simulink model "SixDOFFINAL"  (R2025a)
settings: Solver=FixedStepAuto  StartTime=0.0  StopTime=10  FixedStep=0.001  RelTol=1e-8
PreLoadFcn:
  | P = rocketConfigEuler();
  | assignin('base','P',P);
settings Model: Creator=olive  LastModifiedBy=olivermcnaughton
settings DebuggingCC: UnderSpecifiedDimensionMsg=warning

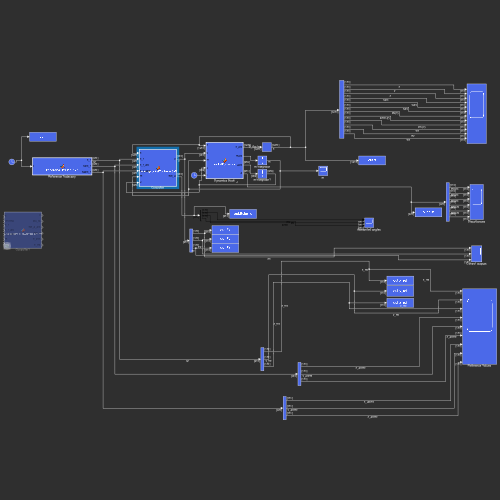
[thumbnail: Simulink's stored preview of the top-level diagram]
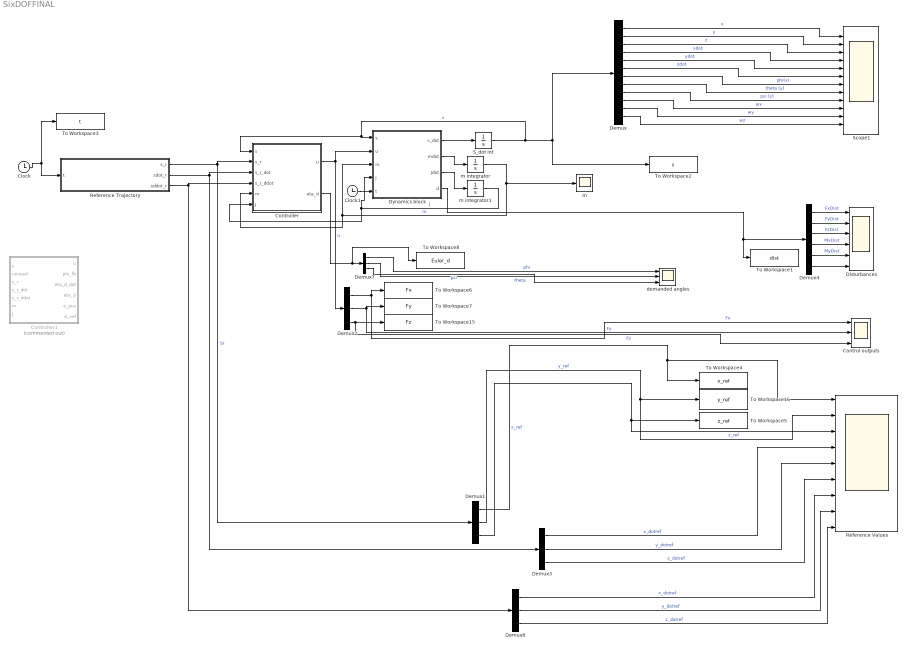
== system SixDOFFINAL ==
  Clock : Clock
  Clock1 : Clock
  Control outputs : Scope  NumInputPorts=3
      settings: ActiveDisplayYMinimum=-27.646396569156394  ActiveDisplayYMaximum=103.07182184101738  DataLoggingVariableName=ScopeData3
  Controller : MATLAB Function  TreatAsAtomicUnit=on
  Controller1 : MATLAB Function  Commented=on  TreatAsAtomicUnit=on
  Demux : Demux  Outputs=12
  Demux{1..3,7..8} (5 alike) : Demux  Outputs=3
  Demux4 : Demux  Outputs=6
  Disturbances : Scope  NumInputPorts=6
      settings: ActiveDisplayYMinimum=-1  ActiveDisplayYMaximum=1
  Dynamics block : MATLAB Function  TreatAsAtomicUnit=on
  Reference Trajectory : MATLAB Function  TreatAsAtomicUnit=on
  Reference Values : Scope  NumInputPorts=9
      settings: ActiveDisplayYMinimum=-0.49999999999999989  ActiveDisplayYMaximum=4.5  DataLoggingVariableName=ScopeData4
  S_dot int : Integrator  InitialCondition=P.init.stateDot
  Scope1 : Scope  NumInputPorts=12
      settings: ActiveDisplayYMinimum=-0.50037904777657061  ActiveDisplayYMaximum=4.5034114299891366
  To Workspace1 : ToWorkspace  VariableName=dist  SaveFormat=Timeseries  SampleTime=-1
  To Workspace15 : ToWorkspace  VariableName=Fz  SaveFormat=Timeseries  SampleTime=-1
  To Workspace16 : ToWorkspace  VariableName=y_ref  SaveFormat=Timeseries  SampleTime=-1
  To Workspace2 : ToWorkspace  VariableName=s  SaveFormat=Timeseries  SampleTime=-1
  To Workspace3 : ToWorkspace  VariableName=t  SaveFormat=Timeseries  SampleTime=-1
  To Workspace4 : ToWorkspace  VariableName=x_ref  SaveFormat=Timeseries  SampleTime=-1
  To Workspace5 : ToWorkspace  VariableName=z_ref  SaveFormat=Timeseries  SampleTime=-1
  To Workspace6 : ToWorkspace  VariableName=Fx  SaveFormat=Timeseries  SampleTime=-1
  To Workspace7 : ToWorkspace  VariableName=Fy  SaveFormat=Timeseries  SampleTime=-1
  To Workspace8 : ToWorkspace  VariableName=Euler_d  SaveFormat=Timeseries  SampleTime=-1
  demanded angles : Scope  NumInputPorts=3
      settings: ActiveDisplayYMinimum=-1  ActiveDisplayYMaximum=1  DataLoggingVariableName=ScopeData5
  m : Scope
      settings: ActiveDisplayYMinimum=23.539410855126405  ActiveDisplayYMaximum=25.162287682763733
  m integrator : Integrator  InitialCondition=P.init.mass
  m integrator1 : Integrator  InitialCondition=P.init.J
  wires:
  Dynamics block/1(s_dot) -> S_dot int/1
  Dynamics block/2(mdot) -> m integrator/1
  Dynamics block/3(Jdot) -> m integrator1/1
  S_dot int/1 -> Controller/1(s), Dynamics block/1(s), To Workspace2/1, Demux/1  "s"
  m integrator1/1 -> Dynamics block/4(J), Controller/6(J)  "J"
  m integrator/1 -> Dynamics block/3(m), Controller/5(m), m/1  "m"
  Demux/1 -> Scope1/1  "x"
  Demux/2 -> Scope1/2  "y"
  Demux/3 -> Scope1/3  "z"
  Demux2/1 -> Control outputs/1, To Workspace6/1  "Fx"
  Controller/1(u) -> Dynamics block/2(u), Demux2/1  "u"
  Clock/1 -> To Workspace3/1, Reference Trajectory/1(t)
  Reference Trajectory/1(s_r) -> Demux1/1, Controller/2(s_r)  "Sr"
  Demux1/2 -> To Workspace16/1, Reference Values/2  "y_ref"
  Demux1/1 -> To Workspace4/1, Reference Values/1  "x_ref"
  Reference Trajectory/2(sdot_r) -> Demux3/1, Controller/3(s_r_dot)
  Clock1/1 -> Dynamics block/5(t)
  Dynamics block/4(d) -> To Workspace1/1, Demux4/1
  Demux1/3 -> To Workspace5/1, Reference Values/3  "z_ref"
  Demux2/2 -> To Workspace7/1, Control outputs/2  "Fy"
  Demux2/3 -> Control outputs/3, To Workspace15/1  "Fz"
  Demux/4 -> Scope1/4  "xdot"
  Demux/5 -> Scope1/5  "ydot"
  Demux/6 -> Scope1/6  "zdot"
  Demux/7 -> Scope1/7  "phi(x)"
  Demux/8 -> Scope1/8  "theta (y)"
  Demux/9 -> Scope1/9  "psi (z)"
  Demux4/1 -> Disturbances/1  "FxDist"
  Demux4/2 -> Disturbances/2  "FyDist"
  Demux4/3 -> Disturbances/3  "FzDist"
  Demux4/4 -> Disturbances/4  "MxDist"
  Demux4/5 -> Disturbances/5  "MyDist"
  Demux4/6 -> Disturbances/6
  Demux7/1 -> demanded angles/1  "phi"
  Demux7/2 -> demanded angles/2  "theta"
  Demux7/3 -> demanded angles/3  "psi"
  Demux/10 -> Scope1/10  "wx"
  Demux/11 -> Scope1/11  "wy"
  Demux/12 -> Scope1/12  "wz"
  Demux3/2 -> Reference Values/5  "y_dotref"
  Demux3/3 -> Reference Values/6  "z_dotref"
  Demux3/1 -> Reference Values/4  "x_dotref"
  Demux8/1 -> Reference Values/7  "x_dotref"
  Demux8/3 -> Reference Values/9  "z_dotref"
  Demux8/2 -> Reference Values/8  "y_dotref"
  Reference Trajectory/3(sddot_r) -> Demux8/1, Controller/4(s_r_ddot)
  Controller/2(eta_d) -> To Workspace8/1, Demux7/1

== matlab function SixDOFFINAL/Reference Trajectory ==
  data: s_r output; sdot_r output; t input; sddot_r output
function [s_r, sdot_r, sddot_r] = trapezoidalRefBlockXYZ(t)
%#codegen
% 3-D trapezoidal reference with smooth polynomial blending between
% acceleration, cruise and deceleration phases – and between consecutive
% motion stages (0→via and via→final).
%
%% 0. Fetch *trajectory* struct once (persistent for speed)
persistent T
if isempty(T)
    % Lock as compile-time constant for codegen
    T = coder.const( rocketConfigEuler().traj );
end
%% 1. Shorthand aliases ----------------------------------------------------
x0=T.x0; xi=T.xi; xf=T.xf;
y0=T.y0; yi=T.yi; yf=T.yf;
z0=T.z0; zi=T.zi; zf=T.zf;
%% ---- 2. Pre-allocate ----------------------------------------------------
s_r     = zeros(3,1);
sdot_r  = zeros(3,1);
sddot_r = zeros(3,1);
% -------------------------------------------------------------------------
% Configure the key-points of the motion here:
% -------------------------------------------------------------------------
%            [x;   y;   z]
 p0 = [x0;    y0;   z0];   % start position
 pi = [xi;    yi;   zi];   % via-point (intermediate target)
 pf = [xf;    yf;   zf];   % final position

 t1=T.t1;  t2=T.t2;
 dt_blend = T.dt_blend;          % polynomial blend window at each transition [s]
 tblend_frac = T.frac_tb;
% -------------------------------------------------------------------------

% Pre-allocate outputs (x,y,z)
 s_r     = zeros(3,1);
 sdot_r  = zeros(3,1);
 sddot_r = zeros(3,1);
% 0b) Step-mode override (any axis) -------------------------------
if T.useStep
    % use initial start pos from your traj struct:
    p0 = [T.x0; T.y0; T.z0];
    % if time < stepTime, stay at p0, else jump to stepTarget
    if t < T.stepTime
        s_r = p0;
    else
        s_r = T.stepTarget;
    end
    sdot_r  = zeros(3,1);
    sddot_r = zeros(3,1);
    return;
end
%=================== 1) Final stop blend (after second stage) =============
 if t >= (t1 + t2 - dt_blend/2)
     t_end = t1 + t2;
     alpha = min((t - (t_end - dt_blend/2)) / dt_blend, 1);
     sigma = 6*alpha^5 - 15*alpha^4 + 10*alpha^3;   % smooth-step 5-th order

     tau2 = t - t1;                                         % local time in stage-2
     [s_pre, sdot_pre, sddot_pre] = localTrapezoidalStage(tau2, pi, pf, t2, dt_blend);

     s_post     = pf;                       % stationary target
     sdot_post  = zeros(3,1);
     sddot_post = zeros(3,1);

     s_r     = (1 - sigma)*s_pre     + sigma*s_post;
     sdot_r  = (1 - sigma)*sdot_pre  + sigma*sdot_post;
     sddot_r = (1 - sigma)*sddot_pre + sigma*sddot_post;
     return;
 end

%=================== 2) Blend between stage-1 and stage-2 =================
 if t > t1 - dt_blend/2 && t < t1 + dt_blend/2
     alpha = (t - (t1 - dt_blend/2)) / dt_blend;
     sigma = 6*alpha^5 - 15*alpha^4 + 10*alpha^3;

     tau1 = t;                 % local time in stage-1
     tau2 = t - t1;            % local time in stage-2

     [s1, sdot1, sddot1] = localTrapezoidalStage(tau1, p0, pi, t1, dt_blend);
     [s2, sdot2, sddot2] = localTrapezoidalStage(tau2, pi, pf, t2, dt_blend);

     s_r     = (1 - sigma)*s1     + sigma*s2;
     sdot_r  = (1 - sigma)*sdot1  + sigma*sdot2;
     sddot_r = (1 - sigma)*sddot1 + sigma*sddot2;
     return;
 end

%=================== 3) Regular evaluation inside one stage ===============
 if t <= t1
     tau = t;   pA = p0;  pB = pi;  tf = t1;
 else
     tau = t - t1;  pA = pi;  pB = pf;  tf = t2;
 end
 [s_r, sdot_r, sddot_r] = localTrapezoidalStage(tau, pA, pB, tf, dt_blend);
end

%=========================================================================
function [s_r, sdot_r, sddot_r] = localTrapezoidalStage(tau, pA, pB, tf, dt_blend) %#codegen
% Vector-form trapezoidal motion with quintic-polynomial blends at the
% cruise boundaries.  Valid for column vectors pA, pB (size = 3×1).

 tb =0.2 * tf;                     % acceleration / deceleration time
 if tb > tf/2;  tb = tf/2;  end
 tc = tf - 2*tb;                    % constant-velocity slice duration

 D   = pB - pA;                     % total displacement (vector)
 den = tb^2 + tb*tc;                % shared denominator
 a   = D / den;                     % constant acceleration (vector)
 V   = a * tb;                      % cruise velocity (vector)

 s_r     = zeros(3,1);
 sdot_r  = zeros(3,1);
 sddot_r = zeros(3,1);

 % ---- 3.1  Acceleration phase ------------------------------------------
 if tau <= tb - dt_blend/2
     sddot_r =  a;
     sdot_r  =  a * tau;
     s_r     =  pA + 0.5*a * tau^2;

 % ---- 3.2  Blend  (acc → cruise) ---------------------------------------
 elseif tau <= tb + dt_blend/2
     tau_b  = tau - (tb - dt_blend/2);
     alpha  = tau_b / dt_blend;
     sigma  = 6*alpha^5 - 15*alpha^4 + 10*alpha^3;

     % edge-A (still accelerating)
     sddot_a = a;
     sdot_a  = a * tau;
     s_a     = pA + 0.5*a * tau^2;

     % edge-C (already at cruise)
     sddot_c = zeros(3,1);
     sdot_c  = V;
     s_c     = pA + 0.5*a * tb^2 + V * (tau - tb);

     s_r     = (1 - sigma).*s_a     + sigma.*s_c;
     sdot_r  = (1 - sigma).*sdot_a  + sigma.*sdot_c;
     sddot_r = (1 - sigma).*sddot_a + sigma.*sddot_c;

 % ---- 3.3  Constant-velocity phase -------------------------------------
 elseif tau <= tb + tc - dt_blend/2
     sddot_r = zeros(3,1);
     sdot_r  = V;
     s_r     = pA + 0.5*a * tb^2 + V * (tau - tb);

 % ---- 3.4  Blend  (cruise → dec) ---------------------------------------
 elseif tau <= tb + tc + dt_blend/2
     tau_b  = tau - (tb + tc - dt_blend/2);
     alpha  = tau_b / dt_blend;
     sigma  = 6*alpha^5 - 15*alpha^4 + 10*alpha^3;

     % edge-C (still cruising)
     sddot_c = zeros(3,1);
     sdot_c  = V;
     s_c     = pA + 0.5*a * tb^2 + V * (tau - tb);

     % edge-D (already decelerating)
     tau2 = tau - (tb + tc);
     p3   = pA + 0.5*a * tb^2 + V * tc;
     sddot_d = -a;
     sdot_d  = V - a * tau2;
     s_d     = p3 + V * tau2 - 0.5*a * tau2.^2;

     s_r     = (1 - sigma).*s_c     + sigma.*s_d;
     sdot_r  = (1 - sigma).*sdot_c  + sigma.*sdot_d;
     sddot_r = (1 - sigma).*sddot_c + sigma.*sddot_d;

 % ---- 3.5  Deceleration phase ------------------------------------------
 else
     tau2 = tau - (tb + tc);
     p3   = pA + 0.5*a * tb^2 + V * tc;
     sddot_r = -a;
     sdot_r  = V - a * tau2;
     s_r     = p3 + V * tau2 - 0.5*a * tau2.^2;
 end
end

== matlab function SixDOFFINAL/Dynamics block ==
  data: s input size=[12,1]; u input; m input; J input; s_dot output size=[12,1]; mdot output size=[1,1]; Jdot output size=[3,3]; t input; d output size=[6,1]
function [s_dot, mdot, Jdot, d] = rocketDynamics(s, u, m, J, t) %#codegen
%ROCKETDYNAMICS  6‑DoF rigid‑body dynamics for a TVC rocket (single nozzle)
%                Disturbance wrench can now be specified in EITHER the
%                body frame or the global (inertial) frame – switchable
%                via flags in rocketConfig.m.
%
%  Inputs / outputs are unchanged from earlier versions.
%  Added parameters (in rocketConfig):
%     useDist            – enable / disable disturbances      (bool)
%     distForceGlobal    – true  → distForceFcn(t) returns GLOBAL‑frame force
%                           false → distForceFcn(t) returns BODY‑frame force
%     distMomentGlobal   – analogous flag for moments
% -------------------------------------------------------------------------

%% 0.  Configuration (read once) -----------------------------------------
persistent P
if isempty(P)
    P = rocketConfigEuler();
    % default missing flags
    if ~isfield(P, 'distForceGlobal');  P.distForceGlobal  = false; end
    if ~isfield(P, 'distMomentGlobal'); P.distMomentGlobal = false; end
end

% Shorthand constants
 g      = P.g;
 rEng   = P.rEng;
 a1     = P.alpha1;
 a2     = P.alpha2;
 beta   = P.beta;

%% 1.  Unpack state  ------------------------------------------------------
phi   = s(7);         % roll   (rad)
theta = s(8);         % pitch  (rad)
psi   = s(9);         % yaw    (rad)

pb = s(10); qb = s(11); rb = s(12);     % body-axis rates
omegaB = [pb; qb; rb];

%% 1a.  Direction-cosine matrices (BODY → GLOBAL and its inverse) --------
cphi = cos(phi);  sphi = sin(phi);
ctheta = cos(theta); stheta = sin(theta);
cpsi = cos(psi);  spsi = sin(psi);

% ZYX sequence :  R_BG = Rz(psi) * Ry(theta) * Rx(phi)
R_BG = [ ctheta*cpsi,                     ctheta*spsi,                     -stheta;
         sphi*stheta*cpsi - cphi*spsi,          sphi*stheta*spsi + cphi*cpsi,          sphi*ctheta;
         cphi*stheta*cpsi + sphi*spsi,          cphi*stheta*spsi - sphi*cpsi,          cphi*ctheta ];
R_GB = R_BG.';    % BODY ← GLOBAL  (transpose because R is orthonormal)
%% 2.  Disturbance wrench -------------------------------------------------
if P.useDist
    Ftmp = P.distForceFcn(t);   % raw output (3×1)
    Mtmp = P.distMomentFcn(t);

    % Convert to BODY frame if necessary
    if P.distForceGlobal
        Fdist = R_GB * Ftmp;
    else
        Fdist = Ftmp;
    end

    if P.distMomentGlobal
        Mdist = R_GB * Mtmp;
    else
        Mdist = Mtmp;
    end
else
    Fdist = zeros(3,1);
    Mdist = zeros(3,1);
end

%% 3.  Control input & mass / inertia decay ------------------------------
% Fbody = u(:);                     % commanded thrust in BODY frame
   %% 3.  Control input & mass / inertia decay ------------------------------
    % decompose the controller’s Fx,Fy,Fz into Fe and gimbals
    Fx = u(1);
    Fy = u(2);
    Fz = u(3);

    % recover gimbal angles (about body-Y for x-tilt, about body-X for y-tilt)
    phi_x = atan2( Fx,  Fz );      % tilt in the X–Z plane
    phi_y = -atan2(Fy,  Fz );      % tilt in the Y–Z plane

    % total thrust magnitude
    Fe = norm([Fx; Fy; Fz]);

    % now reconstruct a *single* gimbaled body-force vector:
    Fbody = [   Fe*sin(phi_x);
              - Fe*cos(phi_x)*sin(phi_y);
                Fe*cos(phi_x)*cos(phi_y) ];
Fe    = norm(Fbody);
mdot  = -a1 * (beta * Fe);
Jdot  = -a2 * (beta * Fe) * eye(3);      % isotropic inertia decay (placeholder)

%% 4.  Net BODY‑frame forces & moments -----------------------------------
Ftot_body = Fbody + Fdist;
Mbody     = cross(rEng, Ftot_body) + Mdist;

%% 5.  Translational & angular acceleration ------------------------------
aGlobal   = R_BG * Ftot_body / m + [0; 0; -g];
omegaDotB = J \ ( Mbody - cross(omegaB, J*omegaB) );

%% 6.  Euler-angle rates  -------------------------------------------------
% Transformation matrix T such that  [phi̇ thetȧ ψ̇]' = T * [p q r]'
T = [ 1,  sphi*tan(theta),   cphi*tan(theta);
      0,  cphi,             -sphi;
      0,  sphi/ctheta,           cphi/ctheta ];

eulerDot = T * omegaB;     % 3×1  (phi̇ thetȧ ψ̇)'

%% 7.  Assemble full state derivative ------------------------------------
% ṡ = [ v(3);  aGlobal(3);  phi̇ thetȧ ψ̇(3);  ω̇(3) ]
s_dot = [ s(4:6) ; aGlobal ; eulerDot ; omegaDotB ];

d = [Fdist; Mdist];    % 6×1  disturbances actually applied
end

== matlab function SixDOFFINAL/Controller1 ==
  settings: updateMethod=DISCRETE
  data: s input; unused input; s_r input; s_r_dot input; s_r_ddot input; m input; J input; u output; phi_fb output; eta_d_dot output; eta_d output; e_pos output; e_vel output
function [u, phi_fb, eta_d_dot, eta_d, e_pos, e_vel] = ...
         SixDoFBacksteprocketControllerSMC_Euler( ...
                 s, ~, s_r, s_r_dot, s_r_ddot, m, J) %#codegen
% SIXDOFBACKSTEPROCKETCONTROLLERSMC_EULER
% 6-DoF back-stepping + SMC TVC controller (Euler Z-Y-X order)
% — instrumented for Fz build-up logging, but code-gen safe.
%
% OUTPUTS
%   u         (3×1) [Fx; Fy; Fz]  — body-frame thrust command
%   phi_fb    (2×1) [gimbalY; gimbalX]  — for logging
%   eta_d_dot (3×1) desired Euler-angle rates
%   eta_d     (3×1) desired Euler angles
%   e_pos     (3×1) position error
%   e_vel     (3×1) velocity error
% -------------------------------------------------------------------------



%% 1. Persistent parameters ----------------------------------------------
persistent P
if isempty(P)
    P = rocketConfigEuler();
end

%% 2. Unpack state and reference vectors ---------------------------------
x      = s(1:3);                          % position [m]
v      = s(4:6);                          % velocity [m/s]
eta    = s(7:9);                          % [phi; theta; psi] [rad]
omegaB = s(10:12);                        % body rates [p; q; r] [rad/s]

x_d  = s_r(:);
v_d  = s_r_dot(:);
a_d  = s_r_ddot(:);

%% 3. Outer-loop inertial-frame force reference ---------------------------
[F_outer, e_pos, e_vel] = outerForces(x, v, x_d, v_d, a_d, m, P);

%% 4. Desired attitude & its derivative ----------------------------------
[eta_d, eta_d_dot] = attitudeReferenceEuler(F_outer, P);

%% 5. Inner attitude loop (also builds Fz debug struct) ------------------
[M_cmd, Fz_inner, dbg] = ...
    attitudeControlEuler(eta, omegaB, eta_d, eta_d_dot, ...
                         J,   P,      e_pos, e_vel, m, a_d);

%% 6. Actuator mapping ----------------------------------------------------
[u, phi_fb, Fz_cmd_final] = actuatorMapping(M_cmd, Fz_inner, P);

%% 7. Log debug signals – simulation-only --------------------------------
dbg.Fz_cmd_final_6dof = Fz_cmd_final;

end % ========== main function ===========================================


%% =======================================================================
%%                        Helper  functions
%% =======================================================================

% -------------------------------------------------------------------------
function [F_outer, e_pos, e_vel] = outerForces(x, v, x_d, v_d, a_d, m, P)
% OUTERFORCES  Position-error sliding surface + back-stepping + SMC

lambda = ensureVec(P.lambdaPosOuter);
k1     = ensureVec(P.kPos1);
k2     = ensureVec(P.kPos2);
etaSmc = ensureVec(P.etaPosOuter);
psiSmc = ensureVec(P.psiPosOuter);

e_pos = x - x_d;
e_vel = v - v_d;
s_pos = e_vel + lambda .* e_pos;

F_bs_out  = m * ( a_d ...
            - (k1 + k2) .* e_vel ...
            -  (k1 .* k2) .* e_pos ) - e_pos;

F_smc_out = -m * etaSmc .* tanh( s_pos ./ psiSmc );

F_outer    = F_bs_out + F_smc_out;
F_outer(3) = F_outer(3) + m * P.g;   % add gravity
end

% -------------------------------------------------------------------------
function g = ensureVec(val)
% ENSUREVEC  Return a 3×1 vector from scalar or 1×3/3×1 input
if isscalar(val)
    g = repmat(val,3,1);
else
    g = val(:);
end
end

% -------------------------------------------------------------------------
function [eta_d, eta_d_dot] = attitudeReferenceEuler(F, P)
% Build desired Euler angles from desired force vector (ZYX convention)

Fx = F(1);  Fy = F(2);  Fz = F(3);

% 1. Raw commands (avoid singularity if Fz ~ 0)
if abs(Fz) < 1e-6
    phi_raw   = 0;
    theta_raw = 0;
else
    phi_raw   =  atan2( Fy,  Fz);   % roll
    theta_raw = atan2(-Fx,  Fz);    % pitch
end

% 2. Tilt limits
tiltMax = deg2rad(7);
phi_d   = max(min(phi_raw,   tiltMax), -tiltMax);
theta_d = max(min(theta_raw, tiltMax), -tiltMax);

% 3. Yaw command (hold zero)
psi_d   = 0;
eta_d   = [phi_d; theta_d; psi_d];

% 4. Low-pass derivative
persistent eta_prev etaDot_prev
if isempty(eta_prev)
    eta_prev    = eta_d;
    etaDot_prev = zeros(3,1);
end

raw_dot   = angleWrap(eta_d - eta_prev) / P.dtCtrl;
eta_d_dot = P.dfilterA * etaDot_prev + (1-P.dfilterA) * raw_dot;

if isfield(P,'etaDotMax')
    eta_d_dot = max(min(eta_d_dot,P.etaDotMax(:)),-P.etaDotMax(:));
end

eta_prev    = eta_d;
etaDot_prev = eta_d_dot;
end

% -------------------------------------------------------------------------
function [M_cmd, Fz_inner, dbg] = attitudeControlEuler( ...
                 eta, omegaB, eta_d, eta_d_dot, J, P, e_pos, e_vel, m, a_d)
% Inner attitude loop (back-stepping + SMC)  **plus** inner position loop
% that generates the required Fz component.

% 1) Euler-angle error & desired body rates ------------------------------
e_ang   = angleWrap(eta - eta_d);
Tinv_d  = TinvZYX(eta_d(1), eta_d(2));
etaDotB = Tinv_d * eta_d_dot;

% 2) Sliding surface -----------------------------------------------------
e_ang_dot = omegaB - etaDotB;
s_att     = e_ang_dot + P.lambdaAtt * e_ang;

% 3) Torques -------------------------------------------------------------
M_bs  = J * ( -(P.kAtt1+P.kAtt2) * e_ang_dot ...
            -  P.kAtt1*P.kAtt2   * e_ang ) - e_ang;
M_smc = -J .* P.etaAtt .* tanh( s_att ./ P.psiAtt );
M_cmd = M_bs + M_smc;

% 4) Inner *position* loop (Z-force build-up) ----------------------------
term_a   =  m * a_d;
term_vel = -m * (P.kPos3 + P.kPos4) .* e_vel;
term_pos = -m * P.kPos3 .* P.kPos4 .* e_pos;
term_pos1= -e_pos;                    % extra BS term

s_pos    = e_vel + P.lambdaPosInner * e_pos;
F_bs_in  = term_a + term_vel + term_pos + term_pos1;
F_smc_in = -m * P.etaPosInner .* tanh( s_pos ./ P.psiPosInner );

F_inner      = F_bs_in + F_smc_in;
F_inner(3)   = F_inner(3) + m * P.g;   % gravity
Fz_inner     = F_inner(3);


end

% -------------------------------------------------------------------------
function [u, phi_fb, Fz_final] = actuatorMapping(M_cmd, Fz_cmd, P)
% Convert moments + vertical force to 3-axis thrust vector command.

L  = -P.rEng(3);          % lever arm (positive)
Fx = -M_cmd(2) / L;
Fy =  M_cmd(1) / L;
Fz =  Fz_cmd;

F_body = [Fx; Fy; Fz];

% Magnitude limiting -----------------------------------------------------
Fe    = norm(F_body);
FeLim = min(max(Fe, P.FeMin), P.FeMax);
F_body = F_body * FeLim / max(Fe, 1e-9);

% Gimbal angles ----------------------------------------------------------
phi_x =  atan2( F_body(1),  F_body(3) );   % about body-Y
phi_y = -atan2( F_body(2),  F_body(3) );   % about body-X
phi_x = min(max(phi_x, -P.gimbalMax), P.gimbalMax);
phi_y = min(max(phi_y, -P.gimbalMax), P.gimbalMax);

% Outputs ----------------------------------------------------------------
Fx_c = min(max(Fx, -90), 90);
Fy_c = min(max(Fy, -90), 90);
Fz_c = min(max(Fz,   0), 500);

u        = [Fx_c; Fy_c; Fz_c];
phi_fb   = [phi_x; phi_y];
Fz_final = Fz_c;
end

% -------------------------------------------------------------------------
function ang = angleWrap(ang)
% Wrap angle(s) to (-pi, pi]
ang = mod(ang + pi, 2*pi) - pi;
end

% -------------------------------------------------------------------------
function Tinv = TinvZYX(phi, theta)
% Inverse Euler-rate mapping  (ZYX order)
ct  = cos(theta);
Tinv = [ 1 0        -sin(theta);
         0 cos(phi)  sin(phi)*ct;
         0 -sin(phi) cos(phi)*ct ] / ct;
end

% -------------------------------------------------------------------------

== matlab function SixDOFFINAL/Controller ==
  settings: updateMethod=DISCRETE
  data: s input; s_r input; s_r_dot input; s_r_ddot input; m input; J input; u output; eta_d output
function [u, eta_d] = ...
         SixDoFBacksteprocketControllerSMC_Euler( ...
                 s, s_r, s_r_dot, s_r_ddot, m, J) %#codegen

% SIXDOFBACKSTEPROCKETCONTROLLERSMC_EULER
% 6-DoF back-stepping + SMC TVC controller (Euler Z-Y-X order)
% — instrumented for Fz build-up logging, but code-gen safe.
%
% OUTPUTS
%   u         (3×1) [Fx; Fy; Fz]  — body-frame thrust command
%   phi_fb    (2×1) [gimbalY; gimbalX]  — for logging
%   eta_d_dot (3×1) desired Euler-angle rates
%   eta_d     (3×1) desired Euler angles
%   e_pos     (3×1) position error
%   e_vel     (3×1) velocity error
% -------------------------------------------------------------------------
%— default definitions so Simulink/Coder always knows sizes & types —
  u          = zeros(3,1);    % 3×1 vector
  phi_fb     = zeros(2,1);    % 2×1 vector
  eta_d_dot  = zeros(3,1);    % 3×1
  eta_d      = zeros(3,1);
  e_pos      = zeros(3,1);
  e_vel      = zeros(3,1);

%% 1. Persistent parameters ----------------------------------------------
persistent P
if isempty(P)
    P = rocketConfigEuler();
end

%% 2. Unpack state and reference vectors ---------------------------------
x      = s(1:3);                        % position [m]
v      = s(4:6);                          % velocity [m/s]
eta    = s(7:9);                          % [phi; theta; psi] [rad]
omegaB = s(10:12);                        % body rates [p; q; r] [rad/s]

x_d  = s_r(:);
v_d  = s_r_dot(:);
a_d  = s_r_ddot(:);

%% 3. Outer-loop inertial-frame force reference ---------------------------
[F_outer, e_pos, e_vel] = outerForces(x, v, x_d, v_d, a_d, m, P);

%% 4. Desired attitude & its derivative ----------------------------------
[eta_d, eta_d_dot] = attitudeReferenceEuler(F_outer, P);

%% 5. Inner attitude loop (also builds Fz debug struct) ------------------
[M_cmd, Fz_inner] = ...
    attitudeControlEuler(eta, omegaB, eta_d, eta_d_dot, ...
                         J,   P,      e_pos, e_vel, m, a_d);

%% 6. Actuator mapping ----------------------------------------------------
u = actuatorMapping(M_cmd, Fz_inner, P);

end % ========== main function ===========================================


%% =======================================================================
%%                        Helper  functions
%% =======================================================================

% -------------------------------------------------------------------------
function [F_outer, e_pos, e_vel] = outerForces(x, v, x_d, v_d, a_d, m, P)
% OUTERFORCES_UNVECTORIZED  Scalar implementation of outerForces
%   Computes each component without vectorized operations.

% Extract scalar gains and parameters
lambda1   = P.lambdaPosOuter(1);
lambda2   = P.lambdaPosOuter(2);
lambda3   = P.lambdaPosOuter(3);

k1_1      = P.kPos1(1);
k1_2      = P.kPos1(2);
k1_3      = P.kPos1(3);

k2_1      = P.kPos2(1);
k2_2      = P.kPos2(2);
k2_3      = P.kPos2(3);

eta1      = P.etaPosOuter;
eta2      = P.etaPosOuter;
eta3      = P.etaPosOuter;

psi1      = P.psiPosOuter(1);
psi2      = P.psiPosOuter(2);
psi3      = P.psiPosOuter(3);

g   = P.g;

% Preallocate outputs
e_pos = zeros(3,1);
e_vel = zeros(3,1);
s_pos = zeros(3,1);
F_bs_out = zeros(3,1);
F_smc_out = zeros(3,1);
F_outer = zeros(3,1);

% Compute scalar errors and sliding surfaces
% Component 1
x1 = x(1); x2 = x(2); x3 = x(3);
v1 = v(1); v2 = v(2); v3 = v(3);
x_d1 = x_d(1); x_d2 = x_d(2); x_d3 = x_d(3);
v_d1 = v_d(1); v_d2 = v_d(2); v_d3 = v_d(3);
a_d1 = a_d(1); a_d2 = a_d(2); a_d3 = a_d(3);

% Position and velocity errors

e_pos(1) = x1 - x_d1;
e_pos(2) = x2 - x_d2;
e_pos(3) = x3 - x_d3;

e_vel(1) = v1 - v_d1;
e_vel(2) = v2 - v_d2;
e_vel(3) = v3 - v_d3;

% Sliding surfaces
s_pos(1) = e_vel(1) + lambda1 * e_pos(1);
s_pos(2) = e_vel(2) + lambda2 * e_pos(2);
s_pos(3) = e_vel(3) + lambda3 * e_pos(3);

% Back-stepping terms
F_bs_out(1) = m * ( a_d1 - (k1_1 + k2_1) * e_vel(1) - (k1_1 * k2_1) * e_pos(1) ) - e_pos(1);
F_bs_out(2) = m * ( a_d2 - (k1_2 + k2_2) * e_vel(2) - (k1_2 * k2_2) * e_pos(2) ) - e_pos(2);
F_bs_out(3) = m * ( a_d3 - (k1_3 + k2_3) * e_vel(3) - (k1_3 * k2_3) * e_pos(3) ) - e_pos(3);

% Sliding-mode terms
F_smc_out(1) = -m * eta1 * tanh( s_pos(1) / psi1 );
F_smc_out(2) = -m * eta2 * tanh( s_pos(2) / psi2 );
F_smc_out(3) = -m * eta3 * tanh( s_pos(3) / psi3 );

% Combine and add gravity
F_outer(1) = F_bs_out(1) + F_smc_out(1);
F_outer(2) = F_bs_out(2) + F_smc_out(2);
F_outer(3) = F_bs_out(3) + F_smc_out(3) + m * g;
end


% -------------------------------------------------------------------------
function g = ensureVec(val)
% ENSUREVEC  Return a 3×1 vector from scalar or 1×3/3×1 input
if isscalar(val)
    g = repmat(val,3,1);
else
    g = val(:);
end
end

% -------------------------------------------------------------------------
function [eta_d, eta_d_dot] = attitudeReferenceEuler(F, P)
% Build desired Euler angles from desired force vector (ZYX convention)

Fx = F(1);  Fy = F(2);  Fz = F(3);

% 1. Raw commands (avoid singularity if Fz ~ 0)
if abs(Fz) < 1e-6
    phi_raw   = 0;
    theta_raw = 0;
else
    phi_raw   =  atan2( Fy,  Fz);   % roll
    theta_raw = -atan2(Fx,  Fz);    % pitch
end

% 2. Tilt limits
tiltMax = deg2rad(7);
phi_d   = max(min(phi_raw,   tiltMax), -tiltMax);
theta_d = max(min(theta_raw, tiltMax), -tiltMax);

% 3. Yaw command (hold zero)
psi_d   = 0;
eta_d   = [phi_d; theta_d; psi_d];

% 4. Low-pass derivative
persistent eta_prev etaDot_prev
if isempty(eta_prev)
    eta_prev    = eta_d;
    etaDot_prev = zeros(3,1);
end

raw_dot   = angleWrap(eta_d - eta_prev) / P.dtCtrl;
eta_d_dot = P.dfilterA * etaDot_prev + (1-P.dfilterA) * raw_dot;

if isfield(P,'etaDotMax')
    eta_d_dot = max(min(eta_d_dot,P.etaDotMax(:)),-P.etaDotMax(:));
end

eta_prev    = eta_d;
etaDot_prev = eta_d_dot;
end

% -------------------------------------------------------------------------
function [M_cmd, Fz_inner] = attitudeControlEuler( ...
    eta, omegaB, eta_d, eta_d_dot, J, P, e_pos, e_vel, m, a_d)
% ATTITUDECONTROLEULER_UNVECTORIZED  Scalar implementation of attitudeControlEuler

% Extract scalar inputs
eta1 = eta(1); eta2 = eta(2); eta3 = eta(3);
omegaB1 = omegaB(1); omegaB2 = omegaB(2); omegaB3 = omegaB(3);
eta_d1 = eta_d(1); eta_d2 = eta_d(2); eta_d3 = eta_d(3);
eta_d_dot1 = eta_d_dot(1); eta_d_dot2 = eta_d_dot(2); eta_d_dot3 = eta_d_dot(3);
e_pos1 = e_pos(1); e_pos2 = e_pos(2); e_pos3 = e_pos(3);
e_vel1 = e_vel(1); e_vel2 = e_vel(2); e_vel3 = e_vel(3);
a_d1 = a_d(1); a_d2 = a_d(2); a_d3 = a_d(3);

% Inertia scalars
J1 = J(1,1);
J2 = J(2,2);
J3 = J(3,3);

% Attitude control gains
lambdaAtt1 = P.lambdaAtt;
lambdaAtt2 = P.lambdaAtt;
lambdaAtt3 = P.lambdaAtt;

kAtt1 = P.kAtt1;
kAtt2 = P.kAtt2;

etaAtt1 = P.etaAtt;
etaAtt2 = P.etaAtt;
etaAtt3 = P.etaAtt;

psiAtt1 = P.psiAtt;
psiAtt2 = P.psiAtt;
psiAtt3 = P.psiAtt;

% Inner position-loop gains

lambdaPosInner3 = P.lambdaPosInner;

kPos3 = P.kPos3;%10
kPos4 = P.kPos4;%10


etaPosInner3 = P.etaPosInner;


psiPosInner3 = P.psiPosInner;

g = P.g;

% 1) Euler-angle error & desired body rates
% Errors per axis
e_ang1 = angleWrap(eta1 - eta_d1);
e_ang2 = angleWrap(eta2 - eta_d2);
e_ang3 = angleWrap(eta3 - eta_d3);

% Desired rates transform
Tinv_d = TinvZYX(eta_d1, eta_d2);
% etaDotB = Tinv_d * eta_d_dot
etaDotB1 = Tinv_d(1,1)*eta_d_dot1 + Tinv_d(1,2)*eta_d_dot2 + Tinv_d(1,3)*eta_d_dot3;
etaDotB2 = Tinv_d(2,1)*eta_d_dot1 + Tinv_d(2,2)*eta_d_dot2 + Tinv_d(2,3)*eta_d_dot3;
etaDotB3 = Tinv_d(3,1)*eta_d_dot1 + Tinv_d(3,2)*eta_d_dot2 + Tinv_d(3,3)*eta_d_dot3;

% 2) Sliding surface for attitude
% Angular velocity error
 e_ang_dot1 = omegaB1 - etaDotB1;
 e_ang_dot2 = omegaB2 - etaDotB2;
 e_ang_dot3 = omegaB3 - etaDotB3;
% Sliding surface
 s_att1 = e_ang_dot1 + lambdaAtt1 * e_ang1;
 s_att2 = e_ang_dot2 + lambdaAtt2 * e_ang2;
 s_att3 = e_ang_dot3 + lambdaAtt3 * e_ang3;

% 3) Torques
% Back-stepping torque
 M_bs1 = J1 * ( -(kAtt1 + kAtt2) * e_ang_dot1 - kAtt1 * kAtt2 * e_ang1 ) - e_ang1;
 M_bs2 = J2 * ( -(kAtt1 + kAtt2) * e_ang_dot2 - kAtt1 * kAtt2 * e_ang2 ) - e_ang2;
 M_bs3 = J3 * ( -(kAtt1 + kAtt2) * e_ang_dot3 - kAtt1 * kAtt2 * e_ang3 ) - e_ang3;
% Sliding-mode torque
 M_smc1 = -J1 * etaAtt1 * tanh( s_att1 / psiAtt1 );
 M_smc2 = -J2 * etaAtt2 * tanh( s_att2 / psiAtt2 );
 M_smc3 = -J3 * etaAtt3 * tanh( s_att3 / psiAtt3 );
% Commanded moment
 M_cmd = [ M_bs1 + M_smc1;  M_bs2 + M_smc2;  M_bs3 + M_smc3 ];

% 4) Inner position loop (Z-force)
% Build each term

 term_a3   = m * a_d3;


 term_vel3 = -m*(kPos4 + kPos3)*e_vel3;


 term_pos3 = -m*kPos3*kPos4*e_pos3;


 term_pos13 = -e_pos3;

% Sliding surface for position

 s_pos3 = e_vel3 + lambdaPosInner3 * e_pos3;

% BS and SMC in Z-loop

 F_bs_in3 = term_a3 + term_vel3 + term_pos3 + term_pos13;


 F_smc_in3 = -m * etaPosInner3 * tanh( s_pos3 / psiPosInner3 );


 F_inner3 = F_bs_in3 + F_smc_in3 + m * g;


% Extract vertical force and pack debug
 Fz_inner = F_inner3;
end

% -------------------------------------------------------------------------
function u = actuatorMapping(M_cmd, Fz_inner, P)
% Convert moments + vertical force to 3-axis thrust vector command.

L  = -P.rEng(3);          % lever arm (positive)
Fx = -M_cmd(2) / L;
Fy =  M_cmd(1) / L;
Fz =  Fz_inner;

%F_body = [Fx; Fy; Fz];

% % Magnitude limiting -----------------------------------------------------
% Fe    = norm(F_body);
% FeLim = min(max(Fe, P.FeMin), P.FeMax);
% F_body = F_body * FeLim / max(Fe, 1e-9);

% Gimbal angles ----------------------------------------------------------
% phi_x =  atan2( F_body(1),  F_body(3) );   % about body-Y
% phi_y = -atan2( F_body(2),  F_body(3) );   % about body-X
% phi_x = min(max(phi_x, -P.gimbalMax), P.gimbalMax);
% phi_y = min(max(phi_y, -P.gimbalMax), P.gimbalMax);

% Outputs ----------------------------------------------------------------
Fx_c = min(max(Fx, -90), 90);
Fy_c = min(max(Fy, -90), 90);
Fz_c = min(max(Fz,   0), 500);

u        = [Fx_c; Fy_c; Fz_c];

end

% -------------------------------------------------------------------------
function ang = angleWrap(ang)
% Wrap angle(s) to (-pi, pi]
ang = mod(ang + pi, 2*pi) - pi;
end

% -------------------------------------------------------------------------
function Tinv = TinvZYX(phi, theta)
% Inverse Euler-rate mapping  (ZYX order)
ct  = cos(theta);
Tinv = [ 1 0        -sin(theta);
         0 cos(phi)  sin(phi)*ct;
         0 -sin(phi) cos(phi)*ct ] / ct;
end
